simulink model "Simulink_sr46579_Roy_Soham"  (R2019a)
settings: Solver=FixedStepAuto  StartTime=0.0  StopTime=0.2  FixedStep=1/fsample  RelTol=1e-3
InitFcn:
  | fs = 20e3;
  | fsample = 20e6;
libraries: powerlib x20, simulink x4
settings Model: Creator=sr46579  LastModifiedBy=sr46579

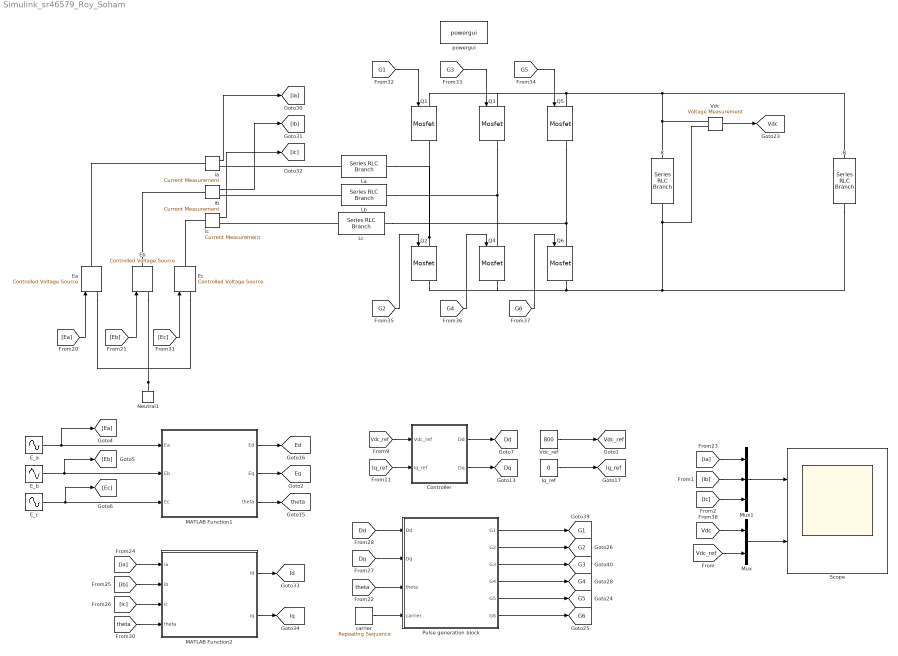
== system Simulink_sr46579_Roy_Soham ==
  C : powerlib/Elements/Series RLC Branch  LConnTagsString=__new0  RConnTagsString=__new0  BranchType=C  Resistance=1  Inductance=1e-3  SetiL0=off  InitialCurrent=0  Capacitance=200e-6  Setx0=on  InitialVoltage=800  Measurements=None
      settings: SourceProductName=Simscape Electrical
  Controller : Subsystem
  E_a : Sin  Amplitude=390  Frequency=2*pi*60  Phase=pi/2  SampleTime=0
  E_b : Sin  Amplitude=390  Frequency=2*pi*60  Phase=(pi/2)-(2*pi/3)  SampleTime=0
  E_c : Sin  Amplitude=390  Frequency=2*pi*60  Phase=(pi/2)+(2*pi/3)  SampleTime=0
  Ea : powerlib/Electrical Sources/Controlled Voltage Source  Initialize=on  Source_Type=AC  Amplitude=0  Phase=0  Frequency=0  Measurements=None
      settings: SourceProductName=Simscape Electrical
  Eb : powerlib/Electrical Sources/Controlled Voltage Source  Initialize=on  Source_Type=AC  Amplitude=0  Phase=0  Frequency=0  Measurements=None
      settings: SourceProductName=Simscape Electrical
  Ec : powerlib/Electrical Sources/Controlled Voltage Source  Initialize=on  Source_Type=AC  Amplitude=0  Phase=0  Frequency=0  Measurements=None
      settings: SourceProductName=Simscape Electrical
  Iq_ref : Constant  Value=0
  La : powerlib/Elements/Series RLC Branch  LConnTagsString=__new0  RConnTagsString=__new0  BranchType=L  Resistance=1  Inductance=20e-3  SetiL0=off  InitialCurrent=0  Capacitance=1e-6  Setx0=off  InitialVoltage=0  Measurements=None
      settings: SourceProductName=Simscape Electrical
  Lb : powerlib/Elements/Series RLC Branch  LConnTagsString=__new0  RConnTagsString=__new0  BranchType=L  Resistance=1  Inductance=20e-3  SetiL0=on  InitialCurrent=0  Capacitance=1e-6  Setx0=off  InitialVoltage=0  Measurements=None
      settings: SourceProductName=Simscape Electrical
  Lc : powerlib/Elements/Series RLC Branch  LConnTagsString=__new0  RConnTagsString=__new0  BranchType=L  Resistance=1  Inductance=20e-3  SetiL0=off  InitialCurrent=0  Capacitance=1e-6  Setx0=off  InitialVoltage=0  Measurements=None
      settings: SourceProductName=Simscape Electrical
  MATLAB Function1 : MATLAB Function  TreatAsAtomicUnit=on
  MATLAB Function2 : MATLAB Function  TreatAsAtomicUnit=on
  Mux : Mux  Inputs=2
  Mux1 : Mux  Inputs=3
  Neutral1 : powerlib/Elements/Neutral  LConnTagsString=a  NodeNumber=1
      settings: SourceProductName=Simscape Electrical  SourceProductBaseCode=PS
  Pulse generation block : Subsystem
  Q{1..6} (6 alike) : powerlib/Power Electronics/Mosfet  Ron=0.1  Lon=0  Rd=0.01  Vfd=0.7  IC=0  Rs=1e5  Cs=inf  Measurements=on
      settings: SourceProductName=Simscape Electrical
  R : powerlib/Elements/Series RLC Branch  LConnTagsString=__new0  RConnTagsString=__new0  BranchType=R  Resistance=100  Inductance=1e-3  SetiL0=off  InitialCurrent=0  Capacitance=1e-6  Setx0=off  InitialVoltage=0  Measurements=None
      settings: SourceProductName=Simscape Electrical
  Scope : Scope  NumInputPorts=2
  Vdc : powerlib/Measurements/Voltage Measurement  PhasorSimulation=off  OutputType=Complex  PSBequivalent=0
      settings: SourceProductName=Simscape Electrical
  Vdc_ref : Constant  Value=800
  carrier : simulink/Sources/Repeating Sequence  rep_seq_t=[0 1/(2*fs) 1/fs]  rep_seq_y=[0 1 0]
  ia : powerlib/Measurements/Current Measurement  PhasorSimulation=off  OutputType=Complex  PSBequivalent=0
      settings: SourceProductName=Simscape Electrical
  ib : powerlib/Measurements/Current Measurement  PhasorSimulation=off  OutputType=Complex  PSBequivalent=0
      settings: SourceProductName=Simscape Electrical
  ic : powerlib/Measurements/Current Measurement  PhasorSimulation=off  OutputType=Complex  PSBequivalent=0
      settings: SourceProductName=Simscape Electrical
  powergui : powerlib/powergui  Priority=1  SimulationMode=Discrete  SampleTime=5e-8  frequency=60  Iterations=50  frequencyindice=0  Pbase=100e6  ErrMax=1e-4  UnitsV=kV  UnitsW=MW  buscounter=0  FunctionMessages=off  echomessages=off  EnableUseOfTLC=off  CurrentSourceSwitches=off  DisableSnubberDevices=off  DisableRonSwitches=off  DisableVfSwitches=off  DisplayEquations=off  AutomaticDiscreteSolvers=off  SolverType=Tustin/Backward Euler (TBE)  Interpol=off  ExternalGateDelay=off  methode=off  Ts=100  x0status=blocks  SPID=off  SwTol=0  HookPort=off  NonlinearTolerance=0  nMaxIteration=15  ContinueOnMaxIteration=off  RestoreLinks=warning  ResistiveCurrentMeasurement=off  Frange=[0:2:500]  Ylog=off  Xlog=on  ShowGrid=off  save=off  variable=ZData  structure=0  ZoomFFT=off  StartTime=0.0  cycles=1  DisplayStyle=1  fundamental=60  FreqAxis=off  MaxFrequency=1000  frequencyindicesteady=1  RmsSteady=1  display=off
      settings: SourceProductName=Simscape Electrical
  tag scope: Dd=global, Dq=global, Ed=global, Eq=global, G1=global, G2=global, G3=global, G4=global, G5=global, G6=global, Id=global, Iq=global, Iq_ref=global, Vdc=global, Vdc_ref=global, theta=global
  wires:
  E_c/1 -> MATLAB Function1/3(Ec), [Ec]
  [Vdc_ref] -> Controller/1(Vdc_ref)
  MATLAB Function1/3(theta) -> [theta]
  E_a/1 -> [Ea], MATLAB Function1/1(Ea)
  [Iq_ref] -> Controller/2(Iq_ref)
  Vdc_ref/1 -> [Vdc_ref]
  E_b/1 -> [Eb], MATLAB Function1/2(Eb)
  Iq_ref/1 -> [Iq_ref]
  MATLAB Function1/2(Eq) -> [Eq]
  MATLAB Function1/1(Ed) -> [Ed]
  Controller/1(Dd) -> [Dd]
  Controller/2(Dq) -> [Dq]
  [ic] -> MATLAB Function2/3(ic)
  [G5] -> Q5/1
  MATLAB Function2/1(Id) -> [Id]
  [Ea] -> Ea/1
  MATLAB Function2/2(Iq) -> [Iq]
  [G6] -> Q6/1
  [Dq] -> Pulse generation block/2(Dq)
  [Dd] -> Pulse generation block/1(Dd)
  [Ec] -> Ec/1
  ib/1 -> [ib]
  [G2] -> Q2/1
  Pulse generation block/3(G3) -> [G3]
  Pulse generation block/1(G1) -> [G1]
  [theta] -> MATLAB Function2/4(theta)
  [G3] -> Q3/1
  Pulse generation block/6(G6) -> [G6]
  carrier/1 -> Pulse generation block/4("carrier ")
  [theta] -> Pulse generation block/3(theta)
  [ia] -> MATLAB Function2/1(ia)
  [Eb] -> Eb/1
  ia/1 -> [ia]
  Pulse generation block/5(G5) -> [G5]
  [G4] -> Q4/1
  [G1] -> Q1/1
  ic/1 -> [ic]
  Pulse generation block/2(G2) -> [G2]
  Vdc/1 -> [Vdc]
  [ib] -> MATLAB Function2/2(ib)
  Pulse generation block/4(G4) -> [G4]
  [ia] -> Mux1/1
  [ib] -> Mux1/2
  [Vdc] -> Mux/1
  Mux/1 -> Scope/2
  [Vdc_ref] -> Mux/2
  Mux1/1 -> Scope/1
  [ic] -> Mux1/3
  connections:
  Q2/LConn1 -- La/RConn1 -- Q1/RConn1
  R/LConn1 -- Q3/LConn1 -- Q1/LConn1 -- Q5/LConn1 -- Vdc/LConn1 -- C/LConn1
  Q6/LConn1 -- Q5/RConn1 -- Lc/RConn1
  Neutral1/LConn1 -- Ec/LConn1 -- Eb/LConn1 -- Ea/LConn1
  Vdc/LConn2 -- R/RConn1 -- Q6/RConn1 -- Q4/RConn1 -- Q2/RConn1 -- C/RConn1
  Q4/LConn1 -- Q3/RConn1 -- Lb/RConn1
  ic/LConn1 -- Ec/RConn1
  ib/LConn1 -- Eb/RConn1
  Lc/LConn1 -- ic/RConn1
  Lb/LConn1 -- ib/RConn1
  ia/LConn1 -- Ea/RConn1
  La/LConn1 -- ia/RConn1

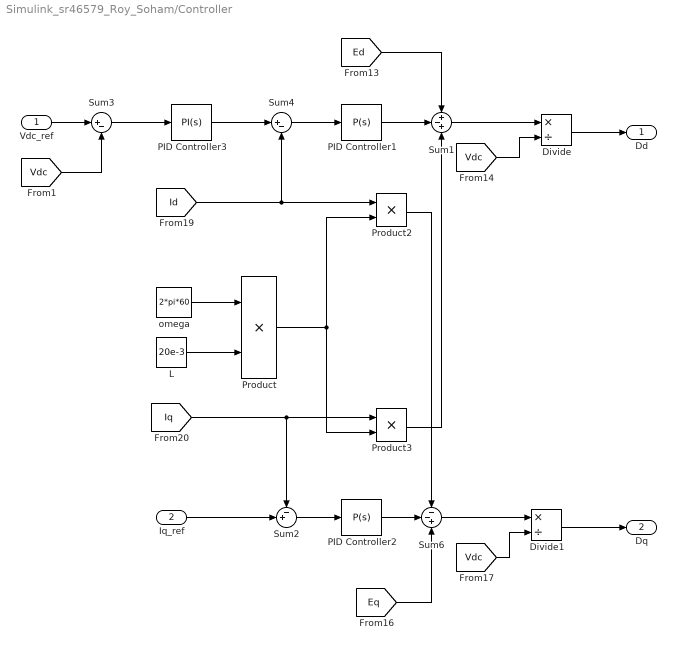
== system Simulink_sr46579_Roy_Soham/Controller ==
  Vdc_ref : Inport
  Iq_ref : Inport  Port=2
  Divide : Product  Inputs=*/
  Divide1 : Product  Inputs=*/
  L : Constant  Value=20e-3
  PID Controller1 : simulink/Continuous/PID Controller  Controller=P  Form=Parallel  TimeDomain=Continuous-time  SampleTime=-1  IntegratorMethod=Forward Euler  FilterMethod=Forward Euler  ControllerParametersSource=internal  P=1000  I=0  D=0  UseFilter=on  N=100  TunerSelectOption=Transfer Function Based (PID Tuner App)  InitialConditionSource=internal  InitialConditionForIntegrator=0  InitialConditionForFilter=0  DifferentiatorICPrevScaledInput=0  ExternalReset=none  TrackingMode=off  Kt=1  LimitOutput=off  UpperSaturationLimit=inf  LowerSaturationLimit=-inf  LinearizeAsGain=on  AntiWindupMode=none  Kb=1  POutMin=[]  POutMax=[]  IOutMin=[]  IOutMax=[]  DOutMin=[]  DOutMax=[]  NOutMin=[]  NOutMax=[]  SumOutMin=[]  SumOutMax=[]  SaturationOutMin=[]  SaturationOutMax=[]  PParamMin=[]  PParamMax=[]  IParamMin=[]  IParamMax=[]  DParamMin=[]  DParamMax=[]  NParamMin=[]  NParamMax=[]  KbParamMin=[]  KbParamMax=[]  KtParamMin=[]  KtParamMax=[]  KbOutMin=[]  KbOutMax=[]  KtOutMin=[]  KtOutMax=[]  IntegratorOutMin=[]  IntegratorOutMax=[]  FilterOutMin=[]  FilterOutMax=[]  SumI1OutMin=[]  SumI1OutMax=[]  SumI2OutMin=[]  SumI2OutMax=[]  SumI3OutMin=[]  SumI3OutMax=[]  SumI4OutMin=[]  SumI4OutMax=[]  SumDOutMin=[]  SumDOutMax=[]  DifferentiatorOutMin=[]  DifferentiatorOutMax=[]  FilterDiffOutCoefMin=[]  FilterDiffOutCoefMax=[]  ReciprocalOutMin=[]  ReciprocalOutMax=[]  SumDenOutMin=[]  SumDenOutMax=[]  SumNumOutMin=[]  SumNumOutMax=[]  DivideOutMin=[]  DivideOutMax=[]  IntegratorContinuousStateAttributes=''  IntegratorStateMustResolveToSignalObject=off  IntegratorRTWStateStorageClass=Auto  FilterContinuousStateAttributes=''  FilterStateMustResolveToSignalObject=off  FilterRTWStateStorageClass=Auto  ParallelPVariant=InternalParameters  IdealPVariant=Disabled  IVariant=Disabled  DVariant=Disabled  IntegratorVariant=Disabled  SatVariant=Disabled  AWVariant=Disabled  PCopyVariant=Disabled  TRVariant=Disabled  FdbkBlocksVariant=Forward  IdealPFdbkVariant=Disabled  SatFdbkVariant=Disabled  DerivativeFilterVariant=Disabled  NVariant=Disabled  NCopyVariant=Disabled_SignalSpec  FilterICVariant=Disabled  IntegratorICVariant=Disabled  ExternalResetVariant=Disabled  TRSumVariant=Passthrough  SumFdbkVariant=Disabled  SumVariant=Passthrough_P
  PID Controller2 : simulink/Continuous/PID Controller  Controller=P  Form=Parallel  TimeDomain=Continuous-time  SampleTime=-1  IntegratorMethod=Forward Euler  FilterMethod=Forward Euler  ControllerParametersSource=internal  P=1000  I=0  D=0  UseFilter=on  N=100  TunerSelectOption=Transfer Function Based (PID Tuner App)  InitialConditionSource=internal  InitialConditionForIntegrator=0  InitialConditionForFilter=0  DifferentiatorICPrevScaledInput=0  ExternalReset=none  TrackingMode=off  Kt=1  LimitOutput=off  UpperSaturationLimit=inf  LowerSaturationLimit=-inf  LinearizeAsGain=on  AntiWindupMode=none  Kb=1  POutMin=[]  POutMax=[]  IOutMin=[]  IOutMax=[]  DOutMin=[]  DOutMax=[]  NOutMin=[]  NOutMax=[]  SumOutMin=[]  SumOutMax=[]  SaturationOutMin=[]  SaturationOutMax=[]  PParamMin=[]  PParamMax=[]  IParamMin=[]  IParamMax=[]  DParamMin=[]  DParamMax=[]  NParamMin=[]  NParamMax=[]  KbParamMin=[]  KbParamMax=[]  KtParamMin=[]  KtParamMax=[]  KbOutMin=[]  KbOutMax=[]  KtOutMin=[]  KtOutMax=[]  IntegratorOutMin=[]  IntegratorOutMax=[]  FilterOutMin=[]  FilterOutMax=[]  SumI1OutMin=[]  SumI1OutMax=[]  SumI2OutMin=[]  SumI2OutMax=[]  SumI3OutMin=[]  SumI3OutMax=[]  SumI4OutMin=[]  SumI4OutMax=[]  SumDOutMin=[]  SumDOutMax=[]  DifferentiatorOutMin=[]  DifferentiatorOutMax=[]  FilterDiffOutCoefMin=[]  FilterDiffOutCoefMax=[]  ReciprocalOutMin=[]  ReciprocalOutMax=[]  SumDenOutMin=[]  SumDenOutMax=[]  SumNumOutMin=[]  SumNumOutMax=[]  DivideOutMin=[]  DivideOutMax=[]  IntegratorContinuousStateAttributes=''  IntegratorStateMustResolveToSignalObject=off  IntegratorRTWStateStorageClass=Auto  FilterContinuousStateAttributes=''  FilterStateMustResolveToSignalObject=off  FilterRTWStateStorageClass=Auto  ParallelPVariant=InternalParameters  IdealPVariant=Disabled  IVariant=Disabled  DVariant=Disabled  IntegratorVariant=Disabled  SatVariant=Disabled  AWVariant=Disabled  PCopyVariant=Disabled  TRVariant=Disabled  FdbkBlocksVariant=Forward  IdealPFdbkVariant=Disabled  SatFdbkVariant=Disabled  DerivativeFilterVariant=Disabled  NVariant=Disabled  NCopyVariant=Disabled_SignalSpec  FilterICVariant=Disabled  IntegratorICVariant=Disabled  ExternalResetVariant=Disabled  TRSumVariant=Passthrough  SumFdbkVariant=Disabled  SumVariant=Passthrough_P
  PID Controller3 : simulink/Continuous/PID Controller  Controller=PI  Form=Parallel  TimeDomain=Continuous-time  SampleTime=-1  IntegratorMethod=Forward Euler  FilterMethod=Forward Euler  ControllerParametersSource=internal  P=0.1  I=10  D=0  UseFilter=on  N=100  TunerSelectOption=Transfer Function Based (PID Tuner App)  InitialConditionSource=internal  InitialConditionForIntegrator=0  InitialConditionForFilter=0  DifferentiatorICPrevScaledInput=0  ExternalReset=none  TrackingMode=off  Kt=1  LimitOutput=off  UpperSaturationLimit=inf  LowerSaturationLimit=-inf  LinearizeAsGain=on  AntiWindupMode=none  Kb=1  POutMin=[]  POutMax=[]  IOutMin=[]  IOutMax=[]  DOutMin=[]  DOutMax=[]  NOutMin=[]  NOutMax=[]  SumOutMin=[]  SumOutMax=[]  SaturationOutMin=[]  SaturationOutMax=[]  PParamMin=[]  PParamMax=[]  IParamMin=[]  IParamMax=[]  DParamMin=[]  DParamMax=[]  NParamMin=[]  NParamMax=[]  KbParamMin=[]  KbParamMax=[]  KtParamMin=[]  KtParamMax=[]  KbOutMin=[]  KbOutMax=[]  KtOutMin=[]  KtOutMax=[]  IntegratorOutMin=[]  IntegratorOutMax=[]  FilterOutMin=[]  FilterOutMax=[]  SumI1OutMin=[]  SumI1OutMax=[]  SumI2OutMin=[]  SumI2OutMax=[]  SumI3OutMin=[]  SumI3OutMax=[]  SumI4OutMin=[]  SumI4OutMax=[]  SumDOutMin=[]  SumDOutMax=[]  DifferentiatorOutMin=[]  DifferentiatorOutMax=[]  FilterDiffOutCoefMin=[]  FilterDiffOutCoefMax=[]  ReciprocalOutMin=[]  ReciprocalOutMax=[]  SumDenOutMin=[]  SumDenOutMax=[]  SumNumOutMin=[]  SumNumOutMax=[]  DivideOutMin=[]  DivideOutMax=[]  IntegratorContinuousStateAttributes=''  IntegratorStateMustResolveToSignalObject=off  IntegratorRTWStateStorageClass=Auto  FilterContinuousStateAttributes=''  FilterStateMustResolveToSignalObject=off  FilterRTWStateStorageClass=Auto  ParallelPVariant=InternalParameters  IdealPVariant=Disabled  IVariant=InternalParameters  DVariant=Disabled  IntegratorVariant=Continuous  SatVariant=Disabled  AWVariant=Passthrough  PCopyVariant=Disabled  TRVariant=Disabled  FdbkBlocksVariant=Forward  IdealPFdbkVariant=Disabled  SatFdbkVariant=Disabled  DerivativeFilterVariant=Disabled  NVariant=Disabled  NCopyVariant=Disabled_SignalSpec  FilterICVariant=Disabled  IntegratorICVariant=InternalICs  ExternalResetVariant=Disabled  TRSumVariant=Passthrough  SumFdbkVariant=Disabled  SumVariant=Sum_PI
  Product : Product
  Product2 : Product
  Product3 : Product
  Sum1 : Sum  Inputs=+-+
  Sum2 : Sum  Inputs=-+|
  Sum3 : Sum  Inputs=|+-
  Sum4 : Sum  Inputs=|+-
  Sum6 : Sum  Inputs=--+
  "omega " : Constant  Value=2*pi*60
  Dd : Outport
  Dq : Outport  Port=2
  wires:
  Product2/1 -> Sum6/1
  [Id] -> Sum4/2, Product2/1
  L/1 -> Product/2
  Divide1/1 -> Dq/1
  [Eq] -> Sum6/3
  [Vdc] -> Divide/2
  Sum6/1 -> Divide1/1
  PID Controller1/1 -> Sum1/2
  Sum1/1 -> Divide/1
  [Ed] -> Sum1/1
  Divide/1 -> Dd/1
  Sum2/1 -> PID Controller2/1
  Product3/1 -> Sum1/3
  PID Controller2/1 -> Sum6/2
  Iq_ref/1 -> Sum2/2
  [Vdc] -> Divide1/2
  Sum4/1 -> PID Controller1/1
  "omega "/1 -> Product/1
  [Iq] -> Sum2/1, Product3/1
  Vdc_ref/1 -> Sum3/1
  [Vdc] -> Sum3/2
  PID Controller3/1 -> Sum4/1
  Sum3/1 -> PID Controller3/1
  Product/1 -> Product2/2, Product3/2

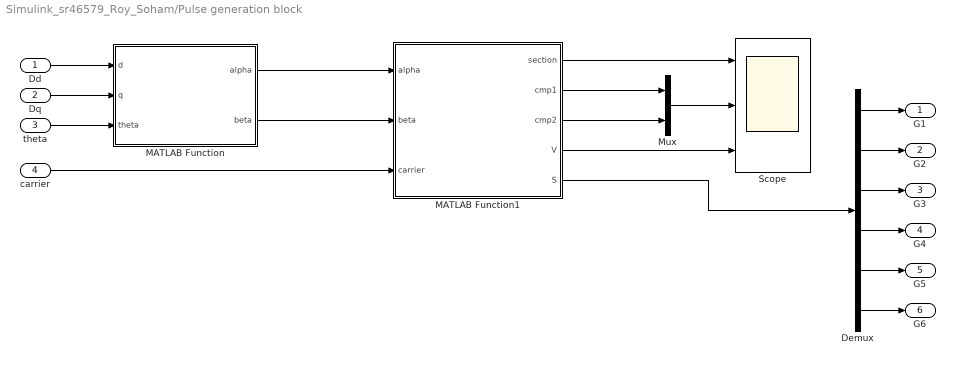
== system Simulink_sr46579_Roy_Soham/Pulse generation block ==
  Dd : Inport
  Dq : Inport  Port=2
  theta : Inport  Port=3
  "carrier " : Inport  Port=4
  Demux : Demux  Outputs=6
  MATLAB Function : MATLAB Function  TreatAsAtomicUnit=on
  MATLAB Function1 : MATLAB Function  TreatAsAtomicUnit=on
  Mux : Mux  Inputs=2
  Scope : Scope  NumInputPorts=3
  G1 : Outport
  G2 : Outport  Port=2
  G3 : Outport  Port=3
  G4 : Outport  Port=4
  G5 : Outport  Port=5
  G6 : Outport  Port=6
  wires:
  MATLAB Function1/3(cmp2) -> Mux/2
  theta/1 -> MATLAB Function/3(theta)
  Dd/1 -> MATLAB Function/1(d)
  Demux/6 -> G6/1
  MATLAB Function1/2(cmp1) -> Mux/1
  MATLAB Function1/4(V) -> Scope/3
  Demux/3 -> G3/1
  MATLAB Function1/1(section) -> Scope/1
  Mux/1 -> Scope/2
  Demux/5 -> G5/1
  Demux/1 -> G1/1
  MATLAB Function1/5(S) -> Demux/1
  Demux/4 -> G4/1
  "carrier "/1 -> MATLAB Function1/3(carrier)
  Dq/1 -> MATLAB Function/2(q)
  Demux/2 -> G2/1
  MATLAB Function/1(alpha) -> MATLAB Function1/1(alpha)
  MATLAB Function/2(beta) -> MATLAB Function1/2(beta)

== matlab function Simulink_sr46579_Roy_Soham/MATLAB Function1 ==
  data: Ed output; Eq output; Ea input; Eb input; theta output; Ec input
function [Ed,Eq,theta]  = abc2dq(Ea,Eb,Ec)

% alpha_beta_gamma domain
E_alpha = sqrt(2/3)*(Ea - (0.5*Eb) - (0.5*Ec));
E_beta = (Eb - Ec)/sqrt(2);

[theta, ~] = cart2pol(E_alpha,E_beta);

% Change range of theta to [0,2*pi]
if theta<0
    theta = theta+2*pi;
end

% dq0 domain
Ed = cos(theta)*E_alpha + sin(theta)*E_beta;
Eq = -sin(theta)*E_alpha + cos(theta)*E_beta;
end

== matlab function Simulink_sr46579_Roy_Soham/MATLAB Function2 ==
  data: Id output; Iq output; ia input; ib input; ic input; theta input
function [Id,Iq]  = abc2dq(ia,ib,ic,theta)

% alpha_beta_gamma domain
i_alpha = sqrt(2/3)*(ia - (0.5*ib) - (0.5*ic));
i_beta = (ib - ic)/sqrt(2);

% dq0 domain
Id = cos(theta)*i_alpha + sin(theta)*i_beta;
Iq = -sin(theta)*i_alpha + cos(theta)*i_beta;
end

== matlab function Simulink_sr46579_Roy_Soham/Pulse generation block/MATLAB Function ==
  data: d input; alpha output; q input; theta input; beta output
function [alpha,beta]= dq2albe(d,q,theta)
alpha = cos(theta)*d - sin(theta)*q;
beta = sin(theta)*d + cos(theta)*q;
end

== matlab function Simulink_sr46579_Roy_Soham/Pulse generation block/MATLAB Function1 ==
  data: alpha input; beta input; section output; cmp1 output; cmp2 output; carrier input; V output; S output
function [section,cmp1,cmp2,V,S] = sv_pwm(alpha,beta,carrier)
[theta, ~] = cart2pol(alpha,beta);

% Change range of theta to [0,2*pi]
if theta<0
    theta = theta+2*pi;
end

section = floor(theta*3/pi)+1;

switch section
    case {1,4}    
        h1 = abs((sqrt(3)*alpha)-beta)/2;
        h2 = abs(beta);
    case {2,5}
        h1 = abs((sqrt(3)*alpha)+beta)/2;
        h2 = abs((sqrt(3)*alpha)-beta)/2;
    otherwise
        h1 = abs(beta);
        h2 = abs((sqrt(3)*alpha)+beta)/2;
end

D1 = sqrt(2)*h1;
D2 = sqrt(2)*h2;

cmp1 = 1-D2;
cmp2 = 1-D1-D2;

if carrier<cmp1 && carrier<cmp2 %V0
    V = [0 0 0];
elseif carrier<cmp1 && carrier>=cmp2 %V1
    switch section
        case 1    
            V = [1 0 0];
        case 2
            V = [1 1 0];
        case 3
            V = [0 1 0];
        case 4
            V = [0 1 1];
        case 5
            V = [0 0 1];
        otherwise
            V = [1 0 1];
    end
else %V2
    switch section
        case 1    
            V = [1 1 0];
        case 2
            V = [0 1 0];
        case 3
            V = [0 1 1];
        case 4
            V = [0 0 1];
        case 5
            V = [1 0 1];
        otherwise
            V = [1 0 0];
    end
end

S1 = V(1);
S2 = not(S1);
S3 = V(2);
S4 = not(S3);
S5 = V(3);
S6 = not(S5);
S = [S1 S2 S3 S4 S5 S6];
end
